simulink model "SprayDryer_DIYcontroller_FOPDT"  (R2018a)
settings: Solver=VariableStepAuto  StartTime=0.0  StopTime=60  FixedStep=0.01  RelTol=1e-3
values from neighbouring files (symbols this model uses):
  ControllerSaturationMax = +10    (= 10)    [CaseStudy2_PID_SprayDryer_DIYcontroller_FOPDT.m]    (also in CaseStudy2_PI_SprayDryer_DIYcontroller_FOPDT.m = inf; CaseStudy3_SprayDryer_with_Heater_DIYcontroller_FOPDT.m = inf)
  ControllerSaturationMin = -10    [CaseStudy2_PID_SprayDryer_DIYcontroller_FOPDT.m]    (also in CaseStudy2_PI_SprayDryer_DIYcontroller_FOPDT.m = -inf; CaseStudy3_SprayDryer_with_Heater_DIYcontroller_FOPDT.m = -inf)
  finalSetpoint = 1    [CaseStudy1_SprayDryer_FOPDT.m]    (also in CaseStudy2_PID_SprayDryer_DIYcontroller_FOPDT.m; CaseStudy2_PI_SprayDryer_DIYcontroller_FOPDT.m; CaseStudy3_SprayDryer_with_Heater_DIYcontroller_FOPDT.m)
  initialSetpoint = 0    [CaseStudy1_SprayDryer_FOPDT.m]    (also in CaseStudy2_PID_SprayDryer_DIYcontroller_FOPDT.m; CaseStudy2_PI_SprayDryer_DIYcontroller_FOPDT.m; CaseStudy3_SprayDryer_with_Heater_DIYcontroller_FOPDT.m)
  K_process = 0.86    [CaseStudy1_SprayDryer_FOPDT.m]    (also in CaseStudy2_PID_SprayDryer_DIYcontroller_FOPDT.m = 2; CaseStudy2_PI_SprayDryer_DIYcontroller_FOPDT.m = 2; CaseStudy3_SprayDryer_with_Heater_DIYcontroller_FOPDT.m = 2)
  kD_controller = kP_controller*tauD_controller    (= 0)    [CaseStudy1_SprayDryer_FOPDT.m]    (also in CaseStudy2_PID_SprayDryer_DIYcontroller_FOPDT.m = kP_controller*tauD_controller; CaseStudy2_PI_SprayDryer_DIYcontroller_FOPDT.m = kP_controller*tauD_controller; CaseStudy3_SprayDryer_with_Heater_DIYcontroller_FOPDT.m)
  kI_controller = kP_controller/tauI_controller    (= 0.504860221536)    [CaseStudy1_SprayDryer_FOPDT.m]    (also in CaseStudy2_PID_SprayDryer_DIYcontroller_FOPDT.m = kP_controller/tauI_controller; CaseStudy2_PI_SprayDryer_DIYcontroller_FOPDT.m = kP_controller/tauI_controller; CaseStudy3_SprayDryer_with_Heater_DIYcontroller_FOPDT.m = 0.02)
  kP_controller = 2.68    [CaseStudy1_SprayDryer_FOPDT.m]    (also in CaseStudy2_PID_SprayDryer_DIYcontroller_FOPDT.m = kPs(j); CaseStudy2_PI_SprayDryer_DIYcontroller_FOPDT.m = kPs(j); CaseStudy3_SprayDryer_with_Heater_DIYcontroller_FOPDT.m = 0.0001)
  tau_process = 2.44    [CaseStudy1_SprayDryer_FOPDT.m]    (also in CaseStudy2_PID_SprayDryer_DIYcontroller_FOPDT.m = 6.8; CaseStudy2_PI_SprayDryer_DIYcontroller_FOPDT.m = 6.8; CaseStudy3_SprayDryer_with_Heater_DIYcontroller_FOPDT.m = 6.8)
  theta_process = 0.16    [CaseStudy1_SprayDryer_FOPDT.m]    (also in CaseStudy2_PID_SprayDryer_DIYcontroller_FOPDT.m = 1; CaseStudy2_PI_SprayDryer_DIYcontroller_FOPDT.m = 1; CaseStudy3_SprayDryer_with_Heater_DIYcontroller_FOPDT.m = 1)
  timeSetpointChange = t_step    [CaseStudy1_SprayDryer_FOPDT.m]    (also in CaseStudy2_PID_SprayDryer_DIYcontroller_FOPDT.m = 10; CaseStudy2_PI_SprayDryer_DIYcontroller_FOPDT.m = 10; CaseStudy3_SprayDryer_with_Heater_DIYcontroller_FOPDT.m = 10)
settings Model: Creator=sadbo  LastModifiedBy=sadbo
settings DataIOCC: SaveFormat=Structure  SaveOutput=off  DSMLogging=off

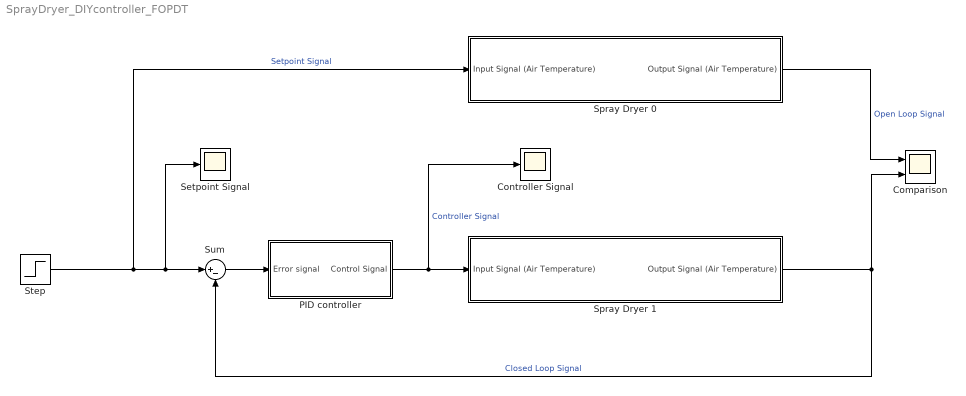
== system SprayDryer_DIYcontroller_FOPDT ==
  "Comparison " : Scope  NumInputPorts=2
  Controller Signal : Scope
  PID controller : Subsystem
  Setpoint Signal : Scope
  "Spray Dryer 0 " : Subsystem
  Spray Dryer 1 : Subsystem
  "Step " : Step  Time=timeSetpointChange  Before=initialSetpoint  After=finalSetpoint  SampleTime=0
  Sum : Sum  Inputs=|+-
  wires:
  Sum/1 -> PID controller/1(Error signal)
  Spray Dryer 1/1("Output Signal (Air Temperature) ") -> "Comparison "/2, Sum/2  "Closed Loop Signal"
  PID controller/1(Control Signal) -> Spray Dryer 1/1(Input Signal (Air Temperature)), Controller Signal/1  "Controller Signal"
  "Spray Dryer 0 "/1("Output Signal (Air Temperature) ") -> "Comparison "/1  "Open Loop Signal"
  "Step "/1 -> "Spray Dryer 0 "/1(Input Signal (Air Temperature)), Setpoint Signal/1, Sum/1  "Setpoint Signal"

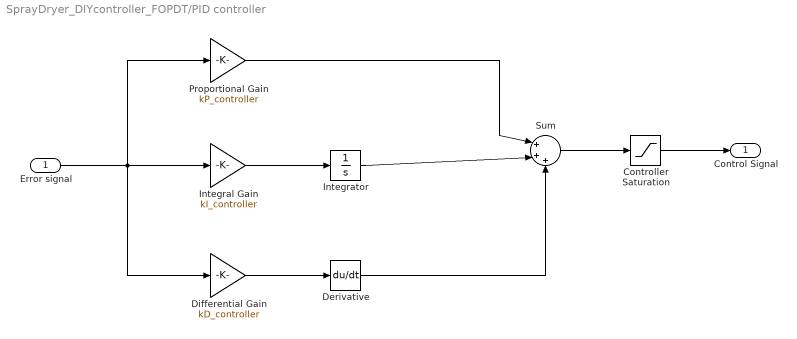
== system SprayDryer_DIYcontroller_FOPDT/PID controller ==
  Error signal : Inport
  Controller Saturation : Saturate  UpperLimit=ControllerSaturationMax  LowerLimit=ControllerSaturationMin
  "Derivative " : Derivative  CoefficientInTFapproximation=+Inf
  Differential Gain : Gain  Gain=kD_controller
  Integral Gain : Gain  Gain=kI_controller
  "Integrator " : Integrator
  Proportional Gain : Gain  Gain=kP_controller
  Sum : Sum  Inputs=|+++
  Control Signal : Outport
  wires:
  Sum/1 -> Controller Saturation/1
  Error signal/1 -> Proportional Gain/1, Integral Gain/1, Differential Gain/1
  Controller Saturation/1 -> Control Signal/1
  Proportional Gain/1 -> Sum/1
  Integral Gain/1 -> "Integrator "/1
  "Integrator "/1 -> Sum/2
  Differential Gain/1 -> "Derivative "/1
  "Derivative "/1 -> Sum/3

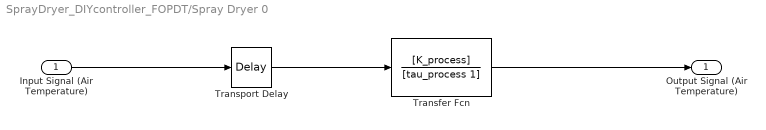
== system SprayDryer_DIYcontroller_FOPDT/Spray Dryer 0  ==
  Input Signal (Air Temperature) : Inport
  Transfer Fcn : TransferFcn  Numerator=[K_process]  Denominator=[tau_process 1]
  Transport Delay : TransportDelay  DelayTime=theta_process
  "Output Signal (Air Temperature) " : Outport
  wires:
  Input Signal (Air Temperature)/1 -> Transport Delay/1
  Transfer Fcn/1 -> "Output Signal (Air Temperature) "/1
  Transport Delay/1 -> Transfer Fcn/1

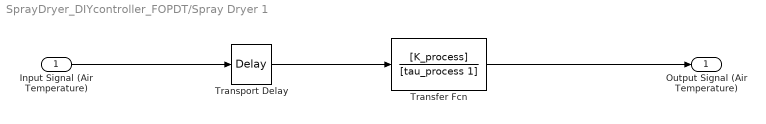
== system SprayDryer_DIYcontroller_FOPDT/Spray Dryer 1 ==
  Input Signal (Air Temperature) : Inport
  Transfer Fcn : TransferFcn  Numerator=[K_process]  Denominator=[tau_process 1]
  Transport Delay : TransportDelay  DelayTime=theta_process
  "Output Signal (Air Temperature) " : Outport
  wires:
  Input Signal (Air Temperature)/1 -> Transport Delay/1
  Transfer Fcn/1 -> "Output Signal (Air Temperature) "/1
  Transport Delay/1 -> Transfer Fcn/1
